simulink model "SEA_dob"  (R2022a)
settings: Solver=FixedStepAuto  StartTime=0.0  StopTime=10  RelTol=1e-3
model workspace (MAT data in the model file):
  Pk = 0
  once = 0
  xk = 0
values from neighbouring files (symbols this model uses):
  de = 0    [params.m]
  dm = 0.0    (= 0)    [estimator.m]    (also in params.m = 0.4)
  Je = 0    [params.m]
  Jm = 0.0104    [estimator.m]    (also in params.m)
  K = 3    [params.m]    (also in rls.m = Pk*Ak.')
  Kd = 0.8    [params.m]
  Ke = block.Dwork(1).Data    [environment.m]    (also in params.m = 25)
  Ki = 0    [params.m]
  Kp = 20    [params.m]
  w2 = 100    [estimator.m]    (also in params.m)
  wc = 10    [estimator.m]    (also in params.m)
libraries: simulink x1, slpidlib x1, ctrlSharedLib x1
settings Model: Creator=mat  LastModifiedBy=mat

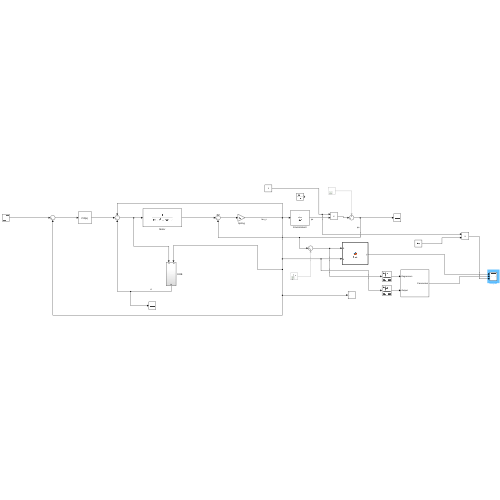
[thumbnail: Simulink's stored preview of the top-level diagram]
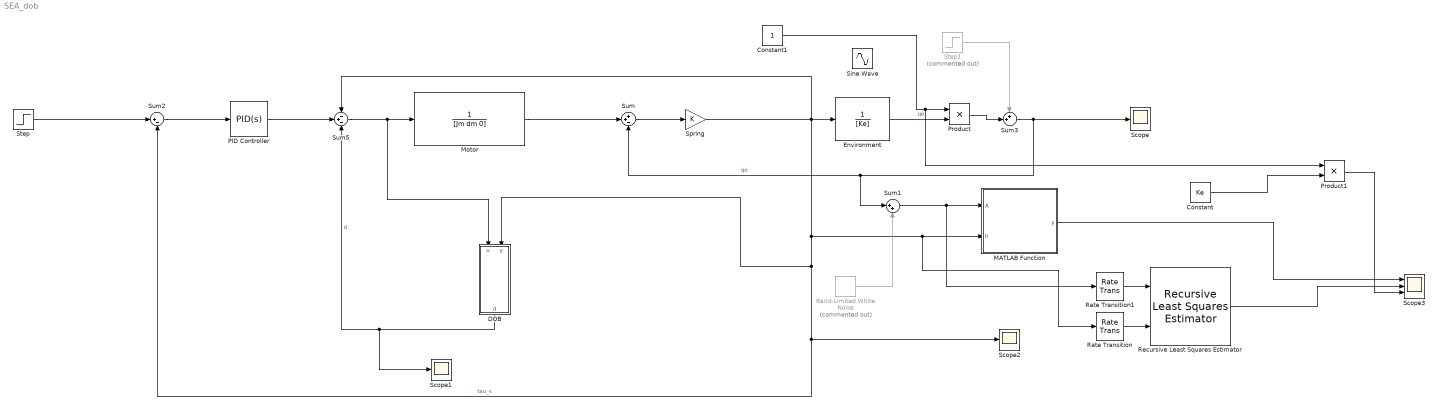
== system SEA_dob ==
  Band-Limited White Noise : simulink/Sources/Band-Limited White Noise  Commented=on  Cov=[0.000001]  Ts=0.001  seed=[23341]
  Constant : Constant  Value=Ke
  Constant1 : Constant
  DOB : Subsystem
  Environment : TransferFcn  Denominator=[Ke]
  MATLAB Function : MATLAB Function  TreatAsAtomicUnit=on  SystemSampleTime=0.001
  Motor : TransferFcn  Denominator=[Jm dm 0]
  PID Controller : slpidlib/PID Controller  Controller=PID  Form=Parallel  TimeDomain=Continuous-time  UseExternalTs=off  SampleTime=-1  IntegratorMethod=Forward Euler  FilterMethod=Forward Euler  ControllerParametersSource=internal  P=Kp  I=Ki  UseKiTs=off  D=Kd  N=100  UseFilter=on  TunerSelectOption=Transfer Function Based (PID Tuner App)  InitialConditionSource=internal  InitialConditionForIntegrator=0  InitialConditionForFilter=0  DifferentiatorICPrevScaledInput=0  ExternalReset=none  TrackingMode=off  Kt=1  LimitOutput=off  SatLimitsSource=internal  UpperSaturationLimit=inf  LowerSaturationLimit=-inf  LinearizeAsGain=on  AntiWindupMode=none  Kb=1  POutMin=[]  POutMax=[]  IOutMin=[]  IOutMax=[]  DOutMin=[]  DOutMax=[]  NOutMin=[]  NOutMax=[]  SumOutMin=[]  SumOutMax=[]  SaturationOutMin=[]  SaturationOutMax=[]  PParamMin=[]  PParamMax=[]  IParamMin=[]  IParamMax=[]  DParamMin=[]  DParamMax=[]  NParamMin=[]  NParamMax=[]  KbParamMin=[]  KbParamMax=[]  KtParamMin=[]  KtParamMax=[]  KbOutMin=[]  KbOutMax=[]  KtOutMin=[]  KtOutMax=[]  IntegratorOutMin=[]  IntegratorOutMax=[]  FilterOutMin=[]  FilterOutMax=[]  SumI1OutMin=[]  SumI1OutMax=[]  SumI2OutMin=[]  SumI2OutMax=[]  SumI3OutMin=[]  SumI3OutMax=[]  SumI4OutMin=[]  SumI4OutMax=[]  SumDOutMin=[]  SumDOutMax=[]  DifferentiatorOutMin=[]  DifferentiatorOutMax=[]  FilterDiffOutCoefMin=[]  FilterDiffOutCoefMax=[]  ReciprocalOutMin=[]  ReciprocalOutMax=[]  SumDenOutMin=[]  SumDenOutMax=[]  SumNumOutMin=[]  SumNumOutMax=[]  DivideOutMin=[]  DivideOutMax=[]  UdiffTsProdOutMin=[]  UdiffTsProdOutMax=[]  NTsProdOutMin=[]  NTsProdOutMax=[]  UintegralTsProdOutMin=[]  UintegralTsProdOutMax=[]  UngainTsProdOutMin=[]  UngainTsProdOutMax=[]  IntegratorContinuousStateAttributes=''  IntegratorStateMustResolveToSignalObject=off  IntegratorRTWStateStorageClass=Auto  FilterContinuousStateAttributes=''  FilterStateMustResolveToSignalObject=off  FilterRTWStateStorageClass=Auto  ParallelPVariant=InternalParameters  IdealPVariant=Disabled  IVariant=InternalParameters  DVariant=InternalParameters  IntegratorVariant=Continuous  SatVariant=Disabled  AWVariant=Passthrough  PCopyVariant=Disabled  TRVariant=Disabled  FdbkBlocksVariant=Forward  IdealPFdbkVariant=Disabled  SatFdbkVariant=Disabled  DerivativeFilterVariant=ContFilter  NVariant=InternalParameters  NCopyVariant=Disabled  FilterICVariant=InternalICsFilter  IntegratorICVariant=InternalICs  ExternalResetVariant=Disabled  TRSumVariant=Passthrough  SumFdbkVariant=Disabled  SumVariant=Sum_PID  TsampFilterVariant=InternalTs  TsampNgainVariant=Passthrough  TsampIntegralVariant=Passthrough  ExternalSaturationOutDataTypeStr=Inherit: Same as second input  aMode=0
  Product : Product
  Product1 : Product
  Rate Transition : RateTransition  OutPortSampleTime=0.001
  Rate Transition1 : RateTransition  OutPortSampleTime=0.001
  Recursive Least Squares Estimator : ctrlSharedLib/Recursive Least Squares Estimator  InitialEstimateSource=None  InitialParameterData=1  P0=1e4  InitialRegressors=0  InitialOutputs=0  History=Infinite  WindowLength=200  EstimationMethod=Forgetting Factor  AdaptationParameter=1  HasTimeVaryingAdaptationParameter=off  NormalizationBias=eps  OutputError=off  OutputP=off  AddEnablePort=off  InputProcessing=Sample-based  Ts=0.001
      settings: SourceProductBaseCode=CT,ID
  Scope : Scope
  Scope1 : Scope
  Scope2 : Scope
  Scope3 : Scope  NumInputPorts=3
  Sine Wave : Sin  Bias=1  SampleTime=0
  Spring : Gain  Gain=K
  Step : Step  SampleTime=0
  Step1 : Step  Commented=on  SampleTime=0
  Sum : Sum  Inputs=++-
  Sum1 : Sum  Inputs=|++
  Sum2 : Sum  Inputs=|+-
  Sum3 : Sum  Inputs=++|
  Sum5 : Sum  Inputs=-+-
  wires:
  Step/1 -> Sum2/1
  Sum2/1 -> PID Controller/1
  Spring/1 -> Sum5/1, Environment/1, Rate Transition/1, MATLAB Function/2(b), Sum2/2, Scope2/1, DOB/2(y)  "tau_s"
  Sum5/1 -> Motor/1, DOB/1(u)
  DOB/1(d) -> Sum5/3, Scope1/1  "d"
  Sum/1 -> Spring/1
  Motor/1 -> Sum/2
  PID Controller/1 -> Sum5/2
  MATLAB Function/1(y) -> Scope3/1
  Sum3/1 -> Sum1/1, Sum/3, Scope/1  "qe"
  Band-Limited White Noise/1 -> Sum1/2
  Step1/1 -> Sum3/1
  Recursive Least Squares Estimator/1 -> Scope3/2
  Rate Transition/1 -> Recursive Least Squares Estimator/2
  Rate Transition1/1 -> Recursive Least Squares Estimator/1
  Product/1 -> Sum3/2
  Environment/1 -> Product/2  "qe"
  Constant/1 -> Product1/2
  Product1/1 -> Scope3/3
  Constant1/1 -> Product1/1, Product/1
  Sum1/1 -> Rate Transition1/1, MATLAB Function/1(A)

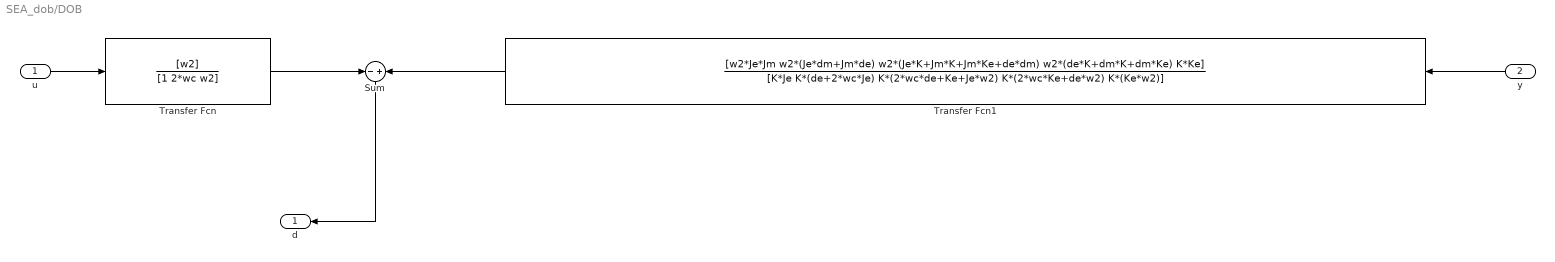
== system SEA_dob/DOB ==
  u : Inport
  y : Inport  Port=2
  Sum : Sum  Inputs=-|+
  Transfer Fcn : TransferFcn  Numerator=[w2]  Denominator=[1 2*wc w2]
  Transfer Fcn1 : TransferFcn  Numerator=[w2*Je*Jm w2*(Je*dm+Jm*de) w2*(Je*K+Jm*K+Jm*Ke+de*dm) w2*(de*K+dm*K+dm*Ke) K*Ke]  Denominator=[K*Je K*(de+2*wc*Je) K*(2*wc*de+Ke+Je*w2) K*(2*wc*Ke+de*w2) K*(Ke*w2)]
  d : Outport
  wires:
  u/1 -> Transfer Fcn/1
  Transfer Fcn1/1 -> Sum/2
  Transfer Fcn/1 -> Sum/1
  y/1 -> Transfer Fcn1/1
  Sum/1 -> d/1

== matlab function SEA_dob/MATLAB Function ==
  data: A input; y output; b input
function y  = RLS(A,b)

persistent once xk Pk;

if isempty(once)
    once = false;
end

if isempty(xk)
    xk = 0;
end

if isempty(Pk)
    Pk = 0;
end

forgetting_factor = 1.0;
Ak = A;
M = size(Ak, 1);

if once    
    Pk = Pk/forgetting_factor;
    % Usare SMW per calcolare Pk
    Pk = Pk - Pk * Ak.' * inv(eye(M) + Ak*Pk*Ak.') * Ak * Pk;
    xk = xk + Pk*Ak.' * (b - Ak*xk);
else
    % Step iniziale (k = 0)
    Pk = inv(Ak.' * Ak);
    xk = (Ak.' * Ak) \ (Ak.' * b);
    if isinf(Pk)
        xk = 0;
        once = false;
    else
        once = true;
    end
end

y = xk;
